simulink subsystem "RX"  (R2022b)
settings: Solver=VariableStepAuto  StartTime=0.0  StopTime=10.0  RelTol=1e-3
settings Model: Creator=Ali-Laptop  LastModifiedBy=Ali-Laptop

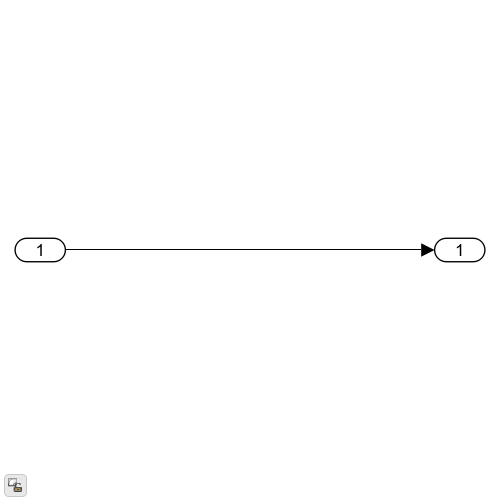
[thumbnail: Simulink's stored preview of the top-level diagram]
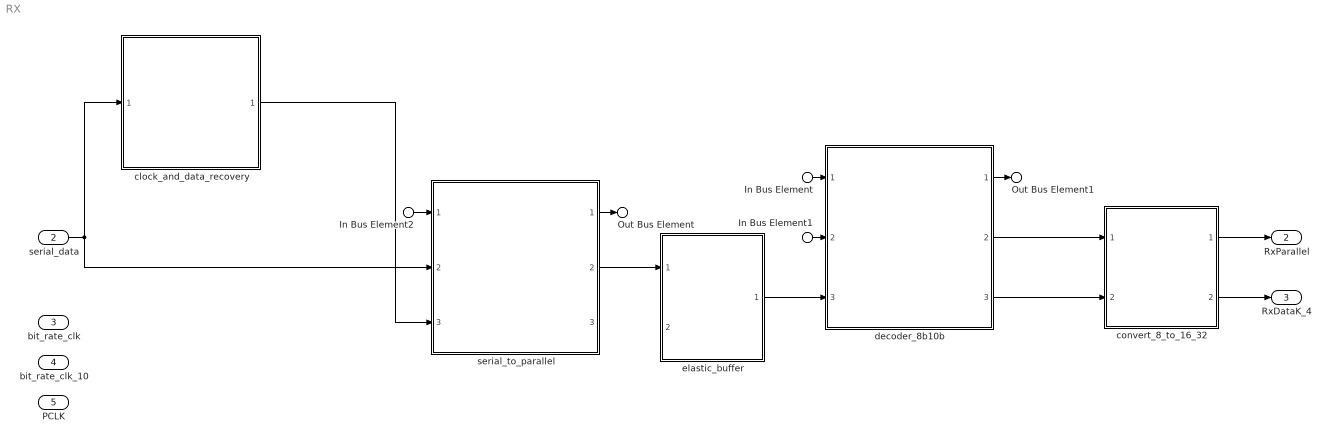
== system RX ==
  In Bus Element : Inport  PortName=digital_out  Element=RxDataK_out
  In Bus Element1 : Inport  PortName=digital_out  Element=RxParallel_8_out
  In Bus Element2 : Inport  PortName=digital_out  Element=RxParallel_10_out
  serial_data : Inport  Port=2
  bit_rate_clk : Inport  Port=3
  bit_rate_clk_10 : Inport  Port=4
  PCLK : Inport  Port=5
  clock_and_data_recovery : Subsystem  ReferencedSubsystem=clock_and_data_recovery
  convert_8_to_16_32 : Subsystem  ReferencedSubsystem=convert_8_to_16_32
  decoder_8b10b : Subsystem  ReferencedSubsystem=decoder_8b10b
  elastic_buffer : Subsystem  ReferencedSubsystem=elastic_buffer
  serial_to_parallel : Subsystem  ReferencedSubsystem=serial_to_parallel
  Out Bus Element : Outport  PortName=digital_in  Element=Serial_in
  Out Bus Element1 : Outport  PortName=digital_in  Element=RxParallel_10_in
  RxParallel : Outport  Port=2
  RxDataK_4 : Outport  Port=3
  wires:
  elastic_buffer/1 -> decoder_8b10b/3
  convert_8_to_16_32/1 -> RxParallel/1
  clock_and_data_recovery/1 -> serial_to_parallel/3
  serial_data/1 -> serial_to_parallel/2, clock_and_data_recovery/1
  serial_to_parallel/1 -> Out Bus Element/1
  In Bus Element2/1 -> serial_to_parallel/1
  decoder_8b10b/1 -> Out Bus Element1/1
  decoder_8b10b/2 -> convert_8_to_16_32/1
  decoder_8b10b/3 -> convert_8_to_16_32/2
  In Bus Element/1 -> decoder_8b10b/1
  In Bus Element1/1 -> decoder_8b10b/2
  convert_8_to_16_32/2 -> RxDataK_4/1
  serial_to_parallel/2 -> elastic_buffer/1
